simulink model "Lab9_Ideal_1"  (R2015a)
settings: Solver=ode5  StartTime=0.0  StopTime=sim_stop_time  FixedStep=sim_step_size  RelTol=1e-3
values from neighbouring files (symbols this model uses):
  Bm = 0.0006001689451    [Lab9.mat]    (also in Lab9_JustinGarcia.m; lab9full.mat)
  Jm = 0.001321184025    [Lab9.mat]    (also in Lab9_JustinGarcia.m; lab9full.mat)
  Kb = 0.4952900056    [Lab9.mat]    (also in Lab9_JustinGarcia.m; lab9full.mat)
  Kt = 0.3233728703    [Lab9.mat]    (also in Lab9_JustinGarcia.m; lab9full.mat)
  Lm = 0.0047    [Lab9.mat]    (also in Lab9_JustinGarcia.m; lab9full.mat)
  Rm = 5.262773292    [Lab9.mat]    (also in Lab9_JustinGarcia.m; lab9full.mat)
  Vref = 9    [Lab9.mat]    (also in Lab9_JustinGarcia.m; lab9full.mat)
settings Model: Creator=009768408  LastModifiedBy=009768408

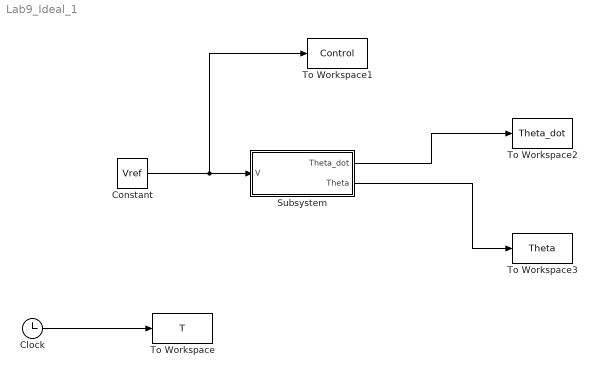
== system Lab9_Ideal_1 ==
  Clock : Clock
  Constant : Constant  Value=Vref
  Subsystem : Subsystem
  To Workspace : ToWorkspace  VariableName=T  SampleTime=-1
  To Workspace1 : ToWorkspace  VariableName=Control  SampleTime=-1
  To Workspace2 : ToWorkspace  VariableName=Theta_dot  SampleTime=-1
  To Workspace3 : ToWorkspace  VariableName=Theta  SampleTime=-1
  wires:
  Clock/1 -> To Workspace/1
  Subsystem/1(Theta_dot) -> To Workspace2/1
  Subsystem/2(Theta) -> To Workspace3/1
  Constant/1 -> To Workspace1/1, Subsystem/1(V)

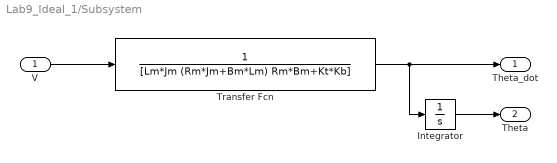
== system Lab9_Ideal_1/Subsystem ==
  V : Inport
  Integrator : Integrator
  Transfer Fcn : TransferFcn  Denominator=[Lm*Jm (Rm*Jm+Bm*Lm) Rm*Bm+Kt*Kb]
  Theta_dot : Outport
  Theta : Outport  Port=2
  wires:
  Integrator/1 -> Theta/1
  Transfer Fcn/1 -> Integrator/1, Theta_dot/1
  V/1 -> Transfer Fcn/1
